simulink model "WER_OBN"  (R2022a)
settings: Solver=ode23tb  StartTime=0.0  StopTime=1.0  RelTol=1e-4  EnableMultiTasking=on
settings Model: Creator=Home  LastModifiedBy=Anastasia
settings SolverCC: AlgebraicLoopSolver=TrustRegion
settings DataIOCC: LimitDataPoints=on  SaveFormat=Array  SignalLoggingSaveFormat=ModelDataLogs  ReturnWorkspaceOutputs=off
settings OptimizationCC: ExpressionDepthLimit=2147483647  InitFltsAndDblsToZero=on  LifeSpan=inf
settings DebuggingCC: SaveWithParameterizedLinksMsg=none  UnderspecifiedInitializationDetection=Classic  MergeDetectMultiDrivingBlocksExec=none  SignalResolutionControl=TryResolveAllWithWarning  SolverPrmCheckMsg=warning  MultiTaskDSMMsg=warning  MultiTaskCondExecSysMsg=none  FcnCallInpInsideContextMsg=warning  UnconnectedInputMsg=warning  UnconnectedOutputMsg=warning  UnconnectedLineMsg=warning  StateNameClashWarn=warning  SFUnexpectedBacktrackingDiag=warning  SFNoUnconditionalDefaultTransitionDiag=warning  SFExecutionAtInitializationDiag=none  SFMachineParentedDataDiag=warning  ArithmeticOperatorsInVariantConditions=warning
settings HardwareCC: ProdBitPerPointer=32  ProdBitPerSizeT=32  ProdBitPerPtrDiffT=32  ProdLargestAtomicFloat=None  ProdIntDivRoundTo=Undefined  ProdEndianess=Unspecified  ProdWordSize=32  ProdHWDeviceType=32-bit Generic
settings ModelReferenceCC: PropagateSignalLabelsOutOfModel=off
settings SFSimCC: SimParseCustomCode=off
settings CodeAppCC: StateflowObjectComments=on
settings GRTTargetCC: TargetFcnLib=ansi_tfl_tmw.mat  TargetLangStandard=C89/C90 (ANSI)  CombineOutputUpdateFcns=off  GRTInterface=on
settings ConfigComp: CovMetricSettings=dw  CovSaveCumulativeToWorkspaceVar=on  CovSaveSingleToWorkspaceVar=on

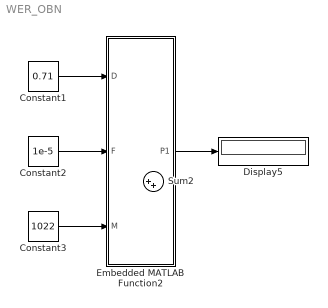
== system WER_OBN ==
  Constant1 : Constant  Value=0.71
  Constant2 : Constant  Value=1e-5
  Constant3 : Constant  Value=1022  VectorParams1D=off
  Display5 : Display
  Embedded MATLAB Function2 : MATLAB Function  TreatAsAtomicUnit=on
  Sum2 : Sum  Inputs=|++
  wires:
  Embedded MATLAB Function2/1(P1) -> Display5/1
  Constant1/1 -> Embedded MATLAB Function2/1(D)
  Constant2/1 -> Embedded MATLAB Function2/2(F)
  Constant3/1 -> Embedded MATLAB Function2/3(M)

== matlab function WER_OBN/Embedded MATLAB Function2 ==
  data: P1 output; D input; F input; M input
function P1= fcn(D,F,M) 
P1=D*(1-F)^(M-1)/(1-(1-D)*(1-F)^(M-1));
end
